simulink model "coif1_7_Level"  (R2021a)
settings: Solver=VariableStepAuto  StartTime=0.0  StopTime=8  RelTol=1e-3
undefined symbols (not defined in the file): lambda2
libraries: dspsigops x15, dspquant2 x1
(part 2 of 4)

== system coif1_7_Level/1st_Level_Decomp/HiD_Even ==
  In_HiD_e : Inport  OutDataTypeStr=double  SampleTime=1/44100
  Add : Sum  AccumDataTypeStr=double  OutDataTypeStr=double  LockScale=on
  Add1 : Sum  AccumDataTypeStr=double  OutDataTypeStr=double  LockScale=on
  Delay{,1..3} (4 alike) : Delay  DelayLength=1  SampleTime=1/44100
  HiD_0 : Constant  Value=0.07273262  OutDataTypeStr=double  SampleTime=1/44100
  HiD_2 : Constant  Value=-0.85257202  OutDataTypeStr=double  SampleTime=1/44100
  HiD_4 : Constant  Value=0.07273262  OutDataTypeStr=double  SampleTime=1/44100
  Multiply : Product  OutDataTypeStr=double  LockScale=on
  Multiply1 : Product  OutDataTypeStr=double  LockScale=on
  Multiply2 : Product  OutDataTypeStr=double  LockScale=on
  Rate Transition : RateTransition  OutPortSampleTime=1/44100
  Rate Transition1 : RateTransition  OutPortSampleTime=1/44100
  Out_HiD_e : Outport  OutDataTypeStr=double  SampleTime=1/44100  VectorParamsAs1DForOutWhenUnconnected=off
  wires:
  In_HiD_e/1 -> Delay/1, Multiply/2
  Delay3/1 -> Add/2
  HiD_2/1 -> Multiply1/1
  Delay/1 -> Rate Transition/1
  Multiply/1 -> Add/1
  Rate Transition/1 -> Delay1/1, Multiply1/2
  HiD_4/1 -> Multiply2/1
  Delay2/1 -> Add1/2
  Multiply1/1 -> Add1/1
  Multiply2/1 -> Delay2/1
  Add1/1 -> Delay3/1
  Rate Transition1/1 -> Multiply2/2
  Add/1 -> Out_HiD_e/1
  Delay1/1 -> Rate Transition1/1
  HiD_0/1 -> Multiply/1

== system coif1_7_Level/1st_Level_Decomp/HiD_Odd ==
  In_HiD_o : Inport  OutDataTypeStr=double  SampleTime=1/44100
  Add : Sum  AccumDataTypeStr=double  OutDataTypeStr=double
  Add1 : Sum  AccumDataTypeStr=double  OutDataTypeStr=double  LockScale=on
  Delay{,1..3} (4 alike) : Delay  DelayLength=1  SampleTime=1/44100
  HiD_1 : Constant  Value=0.337897662  OutDataTypeStr=double  SampleTime=1/44100
  HiD_3 : Constant  Value=0.384864847  OutDataTypeStr=fixdt(1,16,12)  SampleTime=1/44100
  HiD_5 : Constant  Value=-0.015655728  OutDataTypeStr=fixdt(1,16,12)  SampleTime=1/44100
  Multiply : Product  OutDataTypeStr=double  LockScale=on
  Multiply1 : Product  OutDataTypeStr=double  LockScale=on
  Multiply2 : Product  OutDataTypeStr=double  LockScale=on
  Rate Transition : RateTransition  OutPortSampleTime=1/44100
  Rate Transition1 : RateTransition  OutPortSampleTime=1/44100
  Out_HiD_o : Outport  OutDataTypeStr=double  SampleTime=1/44100  VectorParamsAs1DForOutWhenUnconnected=off
  wires:
  In_HiD_o/1 -> Delay/1, Multiply/2
  Delay3/1 -> Add/2
  HiD_3/1 -> Multiply1/1
  Multiply/1 -> Add/1
  Rate Transition/1 -> Delay1/1, Multiply1/2
  Delay2/1 -> Add1/2
  Multiply1/1 -> Add1/1
  Multiply2/1 -> Delay2/1
  Add1/1 -> Delay3/1
  Rate Transition1/1 -> Multiply2/2
  Add/1 -> Out_HiD_o/1
  Delay1/1 -> Rate Transition1/1
  HiD_1/1 -> Multiply/1
  Delay/1 -> Rate Transition/1
  HiD_5/1 -> Multiply2/1

== system coif1_7_Level/1st_Level_Decomp/LoD_Even ==
  In_LoD_e : Inport  OutDataTypeStr=double  SampleTime=1/44100
  Add : Sum  AccumDataTypeStr=double  OutDataTypeStr=double  LockScale=on
  Add1 : Sum  AccumDataTypeStr=double  OutDataTypeStr=double  LockScale=on
  Delay{,1..3} (4 alike) : Delay  DelayLength=1  SampleTime=1/44100
  LoD_0 : Constant  Value=-0.015655728  OutDataTypeStr=double  SampleTime=1/44100
  LoD_2 : Constant  Value=0.384864847  OutDataTypeStr=double  SampleTime=1/44100
  LoD_4 : Constant  Value=0.337897662  OutDataTypeStr=double  SampleTime=1/44100
  Multiply : Product  OutDataTypeStr=double  LockScale=on
  Multiply1 : Product  OutDataTypeStr=double  LockScale=on
  Multiply2 : Product  OutDataTypeStr=double  LockScale=on
  Rate Transition : RateTransition  OutPortSampleTime=1/44100
  Rate Transition1 : RateTransition  OutPortSampleTime=1/44100
  Out_LoD_e : Outport  OutDataTypeStr=double  SampleTime=1/44100  VectorParamsAs1DForOutWhenUnconnected=off
  wires:
  In_LoD_e/1 -> Delay/1, Multiply/2
  Delay3/1 -> Add/2
  LoD_2/1 -> Multiply1/1
  Multiply/1 -> Add/1
  Rate Transition/1 -> Delay1/1, Multiply1/2
  LoD_4/1 -> Multiply2/1
  Delay2/1 -> Add1/2
  Multiply1/1 -> Add1/1
  Multiply2/1 -> Delay2/1
  Add1/1 -> Delay3/1
  Rate Transition1/1 -> Multiply2/2
  Add/1 -> Out_LoD_e/1
  Delay1/1 -> Rate Transition1/1
  LoD_0/1 -> Multiply/1
  Delay/1 -> Rate Transition/1

== system coif1_7_Level/1st_Level_Decomp/LoD_Odd ==
  In_LoD_o : Inport  OutDataTypeStr=double  SampleTime=1/44100
  Add : Sum  AccumDataTypeStr=double  OutDataTypeStr=double  LockScale=on
  Add1 : Sum  AccumDataTypeStr=double  OutDataTypeStr=double  LockScale=on
  Delay{,1..3} (4 alike) : Delay  DelayLength=1  SampleTime=1/44100
  LoD_1 : Constant  Value=-0.07273262  OutDataTypeStr=double  SampleTime=1/44100
  LoD_3 : Constant  Value=0.85257202  OutDataTypeStr=double  SampleTime=1/44100
  LoD_5 : Constant  Value=-0.07273262  OutDataTypeStr=double  SampleTime=1/44100
  Multiply : Product  OutDataTypeStr=double  LockScale=on
  Multiply1 : Product  OutDataTypeStr=double  LockScale=on
  Multiply2 : Product  OutDataTypeStr=double  LockScale=on
  Rate Transition : RateTransition  OutPortSampleTime=1/44100
  Rate Transition1 : RateTransition  OutPortSampleTime=1/44100
  Out_LoD_o : Outport  OutDataTypeStr=double  SampleTime=1/44100  VectorParamsAs1DForOutWhenUnconnected=off
  wires:
  In_LoD_o/1 -> Delay/1, Multiply/2
  Delay3/1 -> Add/2
  LoD_3/1 -> Multiply1/1
  Delay/1 -> Rate Transition/1
  Multiply/1 -> Add/1
  Rate Transition/1 -> Delay1/1, Multiply1/2
  LoD_5/1 -> Multiply2/1
  Delay2/1 -> Add1/2
  Multiply1/1 -> Add1/1
  Multiply2/1 -> Delay2/1
  Add1/1 -> Delay3/1
  Rate Transition1/1 -> Multiply2/2
  Add/1 -> Out_LoD_o/1
  Delay1/1 -> Rate Transition1/1
  LoD_1/1 -> Multiply/1

== system coif1_7_Level/1st_Level_Recon/HiR_Even1 ==
  In_HiR_e : Inport  OutDataTypeStr=double  SampleTime=1/44100
  Add : Sum  AccumDataTypeStr=double  OutDataTypeStr=double  LockScale=on
  Add1 : Sum  AccumDataTypeStr=double  OutDataTypeStr=double  LockScale=on
  Delay{,1..3} (4 alike) : Delay  DelayLength=1  SampleTime=1/44100
  HiR_0 : Constant  Value=-0.015655728  OutDataTypeStr=double  SampleTime=1/44100
  HiR_2 : Constant  Value=0.384864847  OutDataTypeStr=double  SampleTime=1/44100
  HiR_4 : Constant  Value=0.337897662  OutDataTypeStr=double  SampleTime=1/44100
  Multiply : Product  OutDataTypeStr=double  LockScale=on
  Multiply1 : Product  OutDataTypeStr=double  LockScale=on
  Multiply2 : Product  OutDataTypeStr=double  LockScale=on
  Rate Transition : RateTransition  OutPortSampleTime=1/44100
  Rate Transition1 : RateTransition  OutPortSampleTime=1/44100
  Out_HiR_e : Outport  OutDataTypeStr=double  SampleTime=1/44100  VectorParamsAs1DForOutWhenUnconnected=off
  wires:
  In_HiR_e/1 -> Multiply/2, Delay/1
  Delay/1 -> Rate Transition/1
  Delay3/1 -> Add/2
  Multiply/1 -> Add/1
  HiR_0/1 -> Multiply/1
  HiR_2/1 -> Multiply1/1
  Rate Transition/1 -> Delay1/1, Multiply1/2
  Add/1 -> Out_HiR_e/1
  Delay1/1 -> Rate Transition1/1
  Rate Transition1/1 -> Multiply2/2
  Multiply2/1 -> Delay2/1
  Delay2/1 -> Add1/2
  Multiply1/1 -> Add1/1
  Add1/1 -> Delay3/1
  HiR_4/1 -> Multiply2/1

== system coif1_7_Level/1st_Level_Recon/HiR_Odd1 ==
  In_HiR_o : Inport  OutDataTypeStr=double  SampleTime=1/44100
  Add1 : Sum  AccumDataTypeStr=double  OutDataTypeStr=double  LockScale=on
  Add2 : Sum  AccumDataTypeStr=double  OutDataTypeStr=double  LockScale=on
  Delay{1..2,4..5} (4 alike) : Delay  DelayLength=1  SampleTime=1/44100
  HiR_1 : Constant  Value=0.07273262  OutDataTypeStr=double  SampleTime=1/44100
  HiR_3 : Constant  Value=-0.85257202  OutDataTypeStr=double  SampleTime=1/44100
  HiR_5 : Constant  Value=0.07273262  OutDataTypeStr=double  SampleTime=1/44100
  Multiply2 : Product  OutDataTypeStr=double  LockScale=on
  Multiply3 : Product  OutDataTypeStr=double  LockScale=on
  Multiply4 : Product  OutDataTypeStr=double  LockScale=on
  Rate Transition1 : RateTransition  OutPortSampleTime=1/44100
  Rate Transition2 : RateTransition  OutPortSampleTime=1/44100
  Out_HiR_o : Outport  OutDataTypeStr=double  SampleTime=1/44100  VectorParamsAs1DForOutWhenUnconnected=off
  wires:
  HiR_5/1 -> Multiply4/1
  Add1/1 -> Out_HiR_o/1
  Rate Transition2/1 -> Multiply4/2
  Rate Transition1/1 -> Delay2/1, Multiply3/2
  Multiply4/1 -> Delay4/1
  Add2/1 -> Delay5/1
  Multiply3/1 -> Add2/1
  Delay4/1 -> Add2/2
  Multiply2/1 -> Add1/1
  Delay2/1 -> Rate Transition2/1
  In_HiR_o/1 -> Multiply2/2, Delay1/1
  Delay1/1 -> Rate Transition1/1
  Delay5/1 -> Add1/2
  HiR_1/1 -> Multiply2/1
  HiR_3/1 -> Multiply3/1

== system coif1_7_Level/1st_Level_Recon/LoR_Even1 ==
  In_LoR_e : Inport  OutDataTypeStr=double  SampleTime=1/44100
  Add1 : Sum  AccumDataTypeStr=double  OutDataTypeStr=double  LockScale=on
  Add2 : Sum  AccumDataTypeStr=double  OutDataTypeStr=double  LockScale=on
  Delay{1..2,4..5} (4 alike) : Delay  DelayLength=1  SampleTime=1/44100
  LoR_0 : Constant  Value=-0.07273262  OutDataTypeStr=double  SampleTime=1/44100
  LoR_2 : Constant  Value=0.85257202  OutDataTypeStr=double  SampleTime=1/44100
  LoR_4 : Constant  Value=-0.07273262  OutDataTypeStr=double  SampleTime=1/44100
  Multiply2 : Product  OutDataTypeStr=double  LockScale=on
  Multiply3 : Product  OutDataTypeStr=double  LockScale=on
  Multiply4 : Product  OutDataTypeStr=double  LockScale=on
  Rate Transition1 : RateTransition  OutPortSampleTime=1/44100
  Rate Transition2 : RateTransition  OutPortSampleTime=1/44100
  Out_LoR_e : Outport  OutDataTypeStr=double  SampleTime=1/44100  VectorParamsAs1DForOutWhenUnconnected=off
  wires:
  Add2/1 -> Delay5/1
  Delay2/1 -> Rate Transition2/1
  Add1/1 -> Out_LoR_e/1
  Multiply3/1 -> Add2/1
  Delay5/1 -> Add1/2
  Delay1/1 -> Rate Transition1/1
  Multiply2/1 -> Add1/1
  Delay4/1 -> Add2/2
  Multiply4/1 -> Delay4/1
  Rate Transition2/1 -> Multiply4/2
  In_LoR_e/1 -> Multiply2/2, Delay1/1
  Rate Transition1/1 -> Delay2/1, Multiply3/2
  LoR_4/1 -> Multiply4/1
  LoR_2/1 -> Multiply3/1
  LoR_0/1 -> Multiply2/1

== system coif1_7_Level/1st_Level_Recon/LoR_Odd1 ==
  In_LoR_o : Inport  OutDataTypeStr=double  SampleTime=1/44100
  Add1 : Sum  AccumDataTypeStr=double  OutDataTypeStr=double  LockScale=on
  Add2 : Sum  AccumDataTypeStr=double  OutDataTypeStr=double  LockScale=on
  Delay{1..2,4..5} (4 alike) : Delay  DelayLength=1  SampleTime=1/44100
  LoR_1 : Constant  Value=0.337897662  OutDataTypeStr=double  SampleTime=1/44100
  LoR_3 : Constant  Value=0.384864847  OutDataTypeStr=double  SampleTime=1/44100
  LoR_5 : Constant  Value=-0.015655728  OutDataTypeStr=double  SampleTime=1/44100
  Multiply2 : Product  OutDataTypeStr=double  LockScale=on
  Multiply3 : Product  OutDataTypeStr=double  LockScale=on
  Multiply4 : Product  OutDataTypeStr=double  LockScale=on
  Rate Transition1 : RateTransition  OutPortSampleTime=1/44100
  Rate Transition2 : RateTransition  OutPortSampleTime=1/44100
  Out_HiR_o : Outport  OutDataTypeStr=double  SampleTime=1/44100  VectorParamsAs1DForOutWhenUnconnected=off
  wires:
  LoR_5/1 -> Multiply4/1
  In_LoR_o/1 -> Multiply2/2, Delay1/1
  LoR_3/1 -> Multiply3/1
  Delay2/1 -> Rate Transition2/1
  Add2/1 -> Delay5/1
  Multiply3/1 -> Add2/1
  Multiply2/1 -> Add1/1
  Delay4/1 -> Add2/2
  Rate Transition1/1 -> Delay2/1, Multiply3/2
  LoR_1/1 -> Multiply2/1
  Delay5/1 -> Add1/2
  Rate Transition2/1 -> Multiply4/2
  Delay1/1 -> Rate Transition1/1
  Multiply4/1 -> Delay4/1
  Add1/1 -> Out_HiR_o/1

== system coif1_7_Level/2nd_Level_Decomp/HiD_Even ==
  In_HiD_e : Inport  OutDataTypeStr=double  SampleTime=1/44100
  Add : Sum  AccumDataTypeStr=double  OutDataTypeStr=double  LockScale=on
  Add1 : Sum  AccumDataTypeStr=double  OutDataTypeStr=double  LockScale=on
  Delay{,1..3} (4 alike) : Delay  DelayLength=1  SampleTime=1/44100
  HiD_0 : Constant  Value=0.07273262  OutDataTypeStr=double  SampleTime=1/44100
  HiD_2 : Constant  Value=-0.85257202  OutDataTypeStr=double  SampleTime=1/44100
  HiD_4 : Constant  Value=0.07273262  OutDataTypeStr=double  SampleTime=1/44100
  Multiply : Product  OutDataTypeStr=double  LockScale=on
  Multiply1 : Product  OutDataTypeStr=double  LockScale=on
  Multiply2 : Product  OutDataTypeStr=double  LockScale=on
  Rate Transition : RateTransition  OutPortSampleTime=1/44100
  Rate Transition1 : RateTransition  OutPortSampleTime=1/44100
  Out_HiD_e : Outport  OutDataTypeStr=double  SampleTime=1/44100  VectorParamsAs1DForOutWhenUnconnected=off
  wires:
  In_HiD_e/1 -> Delay/1, Multiply/2
  Delay3/1 -> Add/2
  HiD_2/1 -> Multiply1/1
  Delay/1 -> Rate Transition/1
  Multiply/1 -> Add/1
  Rate Transition/1 -> Delay1/1, Multiply1/2
  HiD_4/1 -> Multiply2/1
  Delay2/1 -> Add1/2
  Multiply1/1 -> Add1/1
  Multiply2/1 -> Delay2/1
  Add1/1 -> Delay3/1
  Rate Transition1/1 -> Multiply2/2
  Add/1 -> Out_HiD_e/1
  Delay1/1 -> Rate Transition1/1
  HiD_0/1 -> Multiply/1

== system coif1_7_Level/2nd_Level_Decomp/HiD_Odd ==
  In_HiD_o : Inport  OutDataTypeStr=double  SampleTime=1/44100
  Add : Sum  AccumDataTypeStr=double  OutDataTypeStr=double
  Add1 : Sum  AccumDataTypeStr=double  OutDataTypeStr=double  LockScale=on
  Delay{,1..3} (4 alike) : Delay  DelayLength=1  SampleTime=1/44100
  HiD_1 : Constant  Value=0.337897662  OutDataTypeStr=double  SampleTime=1/44100
  HiD_3 : Constant  Value=0.384864847  OutDataTypeStr=fixdt(1,16,12)  SampleTime=1/44100
  HiD_5 : Constant  Value=-0.015655728  OutDataTypeStr=fixdt(1,16,12)  SampleTime=1/44100
  Multiply : Product  OutDataTypeStr=double  LockScale=on
  Multiply1 : Product  OutDataTypeStr=double  LockScale=on
  Multiply2 : Product  OutDataTypeStr=double  LockScale=on
  Rate Transition : RateTransition  OutPortSampleTime=1/44100
  Rate Transition1 : RateTransition  OutPortSampleTime=1/44100
  Out_HiD_o : Outport  OutDataTypeStr=double  SampleTime=1/44100  VectorParamsAs1DForOutWhenUnconnected=off
  wires:
  In_HiD_o/1 -> Delay/1, Multiply/2
  Delay3/1 -> Add/2
  HiD_3/1 -> Multiply1/1
  Multiply/1 -> Add/1
  Rate Transition/1 -> Delay1/1, Multiply1/2
  Delay2/1 -> Add1/2
  Multiply1/1 -> Add1/1
  Multiply2/1 -> Delay2/1
  Add1/1 -> Delay3/1
  Rate Transition1/1 -> Multiply2/2
  Add/1 -> Out_HiD_o/1
  Delay1/1 -> Rate Transition1/1
  HiD_1/1 -> Multiply/1
  Delay/1 -> Rate Transition/1
  HiD_5/1 -> Multiply2/1

== system coif1_7_Level/2nd_Level_Decomp/LoD_Even ==
  In_LoD_e : Inport  OutDataTypeStr=double  SampleTime=1/44100
  Add : Sum  AccumDataTypeStr=double  OutDataTypeStr=double  LockScale=on
  Add1 : Sum  AccumDataTypeStr=double  OutDataTypeStr=double  LockScale=on
  Delay{,1..3} (4 alike) : Delay  DelayLength=1  SampleTime=1/44100
  LoD_0 : Constant  Value=-0.015655728  OutDataTypeStr=double  SampleTime=1/44100
  LoD_2 : Constant  Value=0.384864847  OutDataTypeStr=double  SampleTime=1/44100
  LoD_4 : Constant  Value=0.337897662  OutDataTypeStr=double  SampleTime=1/44100
  Multiply : Product  OutDataTypeStr=double  LockScale=on
  Multiply1 : Product  OutDataTypeStr=double  LockScale=on
  Multiply2 : Product  OutDataTypeStr=double  LockScale=on
  Rate Transition : RateTransition  OutPortSampleTime=1/44100
  Rate Transition1 : RateTransition  OutPortSampleTime=1/44100
  Out_LoD_e : Outport  OutDataTypeStr=double  SampleTime=1/44100  VectorParamsAs1DForOutWhenUnconnected=off
  wires:
  In_LoD_e/1 -> Delay/1, Multiply/2
  Delay3/1 -> Add/2
  LoD_2/1 -> Multiply1/1
  Multiply/1 -> Add/1
  Rate Transition/1 -> Delay1/1, Multiply1/2
  LoD_4/1 -> Multiply2/1
  Delay2/1 -> Add1/2
  Multiply1/1 -> Add1/1
  Multiply2/1 -> Delay2/1
  Add1/1 -> Delay3/1
  Rate Transition1/1 -> Multiply2/2
  Add/1 -> Out_LoD_e/1
  Delay1/1 -> Rate Transition1/1
  LoD_0/1 -> Multiply/1
  Delay/1 -> Rate Transition/1

== system coif1_7_Level/2nd_Level_Decomp/LoD_Odd ==
  In_LoD_o : Inport  OutDataTypeStr=double  SampleTime=1/44100
  Add : Sum  AccumDataTypeStr=double  OutDataTypeStr=double  LockScale=on
  Add1 : Sum  AccumDataTypeStr=double  OutDataTypeStr=double  LockScale=on
  Delay{,1..3} (4 alike) : Delay  DelayLength=1  SampleTime=1/44100
  LoD_1 : Constant  Value=-0.07273262  OutDataTypeStr=double  SampleTime=1/44100
  LoD_3 : Constant  Value=0.85257202  OutDataTypeStr=double  SampleTime=1/44100
  LoD_5 : Constant  Value=-0.07273262  OutDataTypeStr=double  SampleTime=1/44100
  Multiply : Product  OutDataTypeStr=double  LockScale=on
  Multiply1 : Product  OutDataTypeStr=double  LockScale=on
  Multiply2 : Product  OutDataTypeStr=double  LockScale=on
  Rate Transition : RateTransition  OutPortSampleTime=1/44100
  Rate Transition1 : RateTransition  OutPortSampleTime=1/44100
  Out_LoD_o : Outport  OutDataTypeStr=double  SampleTime=1/44100  VectorParamsAs1DForOutWhenUnconnected=off
  wires:
  In_LoD_o/1 -> Delay/1, Multiply/2
  Delay3/1 -> Add/2
  LoD_3/1 -> Multiply1/1
  Delay/1 -> Rate Transition/1
  Multiply/1 -> Add/1
  Rate Transition/1 -> Delay1/1, Multiply1/2
  LoD_5/1 -> Multiply2/1
  Delay2/1 -> Add1/2
  Multiply1/1 -> Add1/1
  Multiply2/1 -> Delay2/1
  Add1/1 -> Delay3/1
  Rate Transition1/1 -> Multiply2/2
  Add/1 -> Out_LoD_o/1
  Delay1/1 -> Rate Transition1/1
  LoD_1/1 -> Multiply/1

== system coif1_7_Level/2nd_Level_Recon/HiR_Even1 ==
  In_HiR_e : Inport  OutDataTypeStr=double  SampleTime=1/44100
  Add : Sum  AccumDataTypeStr=double  OutDataTypeStr=double  LockScale=on
  Add1 : Sum  AccumDataTypeStr=double  OutDataTypeStr=double  LockScale=on
  Delay{,1..3} (4 alike) : Delay  DelayLength=1  SampleTime=1/44100
  HiR_0 : Constant  Value=-0.015655728  OutDataTypeStr=double  SampleTime=1/44100
  HiR_2 : Constant  Value=0.384864847  OutDataTypeStr=double  SampleTime=1/44100
  HiR_4 : Constant  Value=0.337897662  OutDataTypeStr=double  SampleTime=1/44100
  Multiply : Product  OutDataTypeStr=double  LockScale=on
  Multiply1 : Product  OutDataTypeStr=double  LockScale=on
  Multiply2 : Product  OutDataTypeStr=double  LockScale=on
  Rate Transition : RateTransition  OutPortSampleTime=1/44100
  Rate Transition1 : RateTransition  OutPortSampleTime=1/44100
  Out_HiR_e : Outport  OutDataTypeStr=double  SampleTime=1/44100  VectorParamsAs1DForOutWhenUnconnected=off
  wires:
  In_HiR_e/1 -> Multiply/2, Delay/1
  Delay/1 -> Rate Transition/1
  Delay3/1 -> Add/2
  Multiply/1 -> Add/1
  HiR_0/1 -> Multiply/1
  HiR_2/1 -> Multiply1/1
  Rate Transition/1 -> Delay1/1, Multiply1/2
  Add/1 -> Out_HiR_e/1
  Delay1/1 -> Rate Transition1/1
  Rate Transition1/1 -> Multiply2/2
  Multiply2/1 -> Delay2/1
  Delay2/1 -> Add1/2
  Multiply1/1 -> Add1/1
  Add1/1 -> Delay3/1
  HiR_4/1 -> Multiply2/1

== system coif1_7_Level/2nd_Level_Recon/HiR_Odd1 ==
  In_HiR_o : Inport  OutDataTypeStr=double  SampleTime=1/44100
  Add1 : Sum  AccumDataTypeStr=double  OutDataTypeStr=double  LockScale=on
  Add2 : Sum  AccumDataTypeStr=double  OutDataTypeStr=double  LockScale=on
  Delay{1..2,4..5} (4 alike) : Delay  DelayLength=1  SampleTime=1/44100
  HiR_1 : Constant  Value=0.07273262  OutDataTypeStr=double  SampleTime=1/44100
  HiR_3 : Constant  Value=-0.85257202  OutDataTypeStr=double  SampleTime=1/44100
  HiR_5 : Constant  Value=0.07273262  OutDataTypeStr=double  SampleTime=1/44100
  Multiply2 : Product  OutDataTypeStr=double  LockScale=on
  Multiply3 : Product  OutDataTypeStr=double  LockScale=on
  Multiply4 : Product  OutDataTypeStr=double  LockScale=on
  Rate Transition1 : RateTransition  OutPortSampleTime=1/44100
  Rate Transition2 : RateTransition  OutPortSampleTime=1/44100
  Out_HiR_o : Outport  OutDataTypeStr=double  SampleTime=1/44100  VectorParamsAs1DForOutWhenUnconnected=off
  wires:
  HiR_5/1 -> Multiply4/1
  Add1/1 -> Out_HiR_o/1
  Rate Transition2/1 -> Multiply4/2
  Rate Transition1/1 -> Delay2/1, Multiply3/2
  Multiply4/1 -> Delay4/1
  Add2/1 -> Delay5/1
  Multiply3/1 -> Add2/1
  Delay4/1 -> Add2/2
  Multiply2/1 -> Add1/1
  Delay2/1 -> Rate Transition2/1
  In_HiR_o/1 -> Multiply2/2, Delay1/1
  Delay1/1 -> Rate Transition1/1
  Delay5/1 -> Add1/2
  HiR_1/1 -> Multiply2/1
  HiR_3/1 -> Multiply3/1

== system coif1_7_Level/2nd_Level_Recon/LoR_Even1 ==
  In_LoR_e : Inport  OutDataTypeStr=double  SampleTime=1/44100
  Add1 : Sum  AccumDataTypeStr=double  OutDataTypeStr=double  LockScale=on
  Add2 : Sum  AccumDataTypeStr=double  OutDataTypeStr=double  LockScale=on
  Delay{1..2,4..5} (4 alike) : Delay  DelayLength=1  SampleTime=1/44100
  LoR_0 : Constant  Value=-0.07273262  OutDataTypeStr=double  SampleTime=1/44100
  LoR_2 : Constant  Value=0.85257202  OutDataTypeStr=double  SampleTime=1/44100
  LoR_4 : Constant  Value=-0.07273262  OutDataTypeStr=double  SampleTime=1/44100
  Multiply2 : Product  OutDataTypeStr=double  LockScale=on
  Multiply3 : Product  OutDataTypeStr=double  LockScale=on
  Multiply4 : Product  OutDataTypeStr=double  LockScale=on
  Rate Transition1 : RateTransition  OutPortSampleTime=1/44100
  Rate Transition2 : RateTransition  OutPortSampleTime=1/44100
  Out_LoR_e : Outport  OutDataTypeStr=double  SampleTime=1/44100  VectorParamsAs1DForOutWhenUnconnected=off
  wires:
  Add2/1 -> Delay5/1
  Delay2/1 -> Rate Transition2/1
  Add1/1 -> Out_LoR_e/1
  Multiply3/1 -> Add2/1
  Delay5/1 -> Add1/2
  Delay1/1 -> Rate Transition1/1
  Multiply2/1 -> Add1/1
  Delay4/1 -> Add2/2
  Multiply4/1 -> Delay4/1
  Rate Transition2/1 -> Multiply4/2
  In_LoR_e/1 -> Multiply2/2, Delay1/1
  Rate Transition1/1 -> Delay2/1, Multiply3/2
  LoR_4/1 -> Multiply4/1
  LoR_2/1 -> Multiply3/1
  LoR_0/1 -> Multiply2/1

== system coif1_7_Level/2nd_Level_Recon/LoR_Odd1 ==
  In_LoR_o : Inport  OutDataTypeStr=double  SampleTime=1/44100
  Add1 : Sum  AccumDataTypeStr=double  OutDataTypeStr=double  LockScale=on
  Add2 : Sum  AccumDataTypeStr=double  OutDataTypeStr=double  LockScale=on
  Delay{1..2,4..5} (4 alike) : Delay  DelayLength=1  SampleTime=1/44100
  LoR_1 : Constant  Value=0.337897662  OutDataTypeStr=double  SampleTime=1/44100
  LoR_3 : Constant  Value=0.384864847  OutDataTypeStr=double  SampleTime=1/44100
  LoR_5 : Constant  Value=-0.015655728  OutDataTypeStr=double  SampleTime=1/44100
  Multiply2 : Product  OutDataTypeStr=double  LockScale=on
  Multiply3 : Product  OutDataTypeStr=double  LockScale=on
  Multiply4 : Product  OutDataTypeStr=double  LockScale=on
  Rate Transition1 : RateTransition  OutPortSampleTime=1/44100
  Rate Transition2 : RateTransition  OutPortSampleTime=1/44100
  Out_HiR_o : Outport  OutDataTypeStr=double  SampleTime=1/44100  VectorParamsAs1DForOutWhenUnconnected=off
  wires:
  LoR_5/1 -> Multiply4/1
  In_LoR_o/1 -> Multiply2/2, Delay1/1
  LoR_3/1 -> Multiply3/1
  Delay2/1 -> Rate Transition2/1
  Add2/1 -> Delay5/1
  Multiply3/1 -> Add2/1
  Multiply2/1 -> Add1/1
  Delay4/1 -> Add2/2
  Rate Transition1/1 -> Delay2/1, Multiply3/2
  LoR_1/1 -> Multiply2/1
  Delay5/1 -> Add1/2
  Rate Transition2/1 -> Multiply4/2
  Delay1/1 -> Rate Transition1/1
  Multiply4/1 -> Delay4/1
  Add1/1 -> Out_HiR_o/1

== system coif1_7_Level/3rd_Level_Decomp/HiD_Even ==
  In_HiD_e : Inport  OutDataTypeStr=double  SampleTime=1/44100
  Add : Sum  AccumDataTypeStr=double  OutDataTypeStr=double  LockScale=on
  Add1 : Sum  AccumDataTypeStr=double  OutDataTypeStr=double  LockScale=on
  Delay{,1..3} (4 alike) : Delay  DelayLength=1  SampleTime=1/44100
  HiD_0 : Constant  Value=0.07273262  OutDataTypeStr=double  SampleTime=1/44100
  HiD_2 : Constant  Value=-0.85257202  OutDataTypeStr=double  SampleTime=1/44100
  HiD_4 : Constant  Value=0.07273262  OutDataTypeStr=double  SampleTime=1/44100
  Multiply : Product  OutDataTypeStr=double  LockScale=on
  Multiply1 : Product  OutDataTypeStr=double  LockScale=on
  Multiply2 : Product  OutDataTypeStr=double  LockScale=on
  Rate Transition : RateTransition  OutPortSampleTime=1/44100
  Rate Transition1 : RateTransition  OutPortSampleTime=1/44100
  Out_HiD_e : Outport  OutDataTypeStr=double  SampleTime=1/44100  VectorParamsAs1DForOutWhenUnconnected=off
  wires:
  In_HiD_e/1 -> Delay/1, Multiply/2
  Delay3/1 -> Add/2
  HiD_2/1 -> Multiply1/1
  Delay/1 -> Rate Transition/1
  Multiply/1 -> Add/1
  Rate Transition/1 -> Delay1/1, Multiply1/2
  HiD_4/1 -> Multiply2/1
  Delay2/1 -> Add1/2
  Multiply1/1 -> Add1/1
  Multiply2/1 -> Delay2/1
  Add1/1 -> Delay3/1
  Rate Transition1/1 -> Multiply2/2
  Add/1 -> Out_HiD_e/1
  Delay1/1 -> Rate Transition1/1
  HiD_0/1 -> Multiply/1

== system coif1_7_Level/3rd_Level_Decomp/HiD_Odd ==
  In_HiD_o : Inport  OutDataTypeStr=double  SampleTime=1/44100
  Add : Sum  AccumDataTypeStr=double  OutDataTypeStr=double
  Add1 : Sum  AccumDataTypeStr=double  OutDataTypeStr=double  LockScale=on
  Delay{,1..3} (4 alike) : Delay  DelayLength=1  SampleTime=1/44100
  HiD_1 : Constant  Value=0.337897662  OutDataTypeStr=double  SampleTime=1/44100
  HiD_3 : Constant  Value=0.384864847  OutDataTypeStr=fixdt(1,16,12)  SampleTime=1/44100
  HiD_5 : Constant  Value=-0.015655728  OutDataTypeStr=fixdt(1,16,12)  SampleTime=1/44100
  Multiply : Product  OutDataTypeStr=double  LockScale=on
  Multiply1 : Product  OutDataTypeStr=double  LockScale=on
  Multiply2 : Product  OutDataTypeStr=double  LockScale=on
  Rate Transition : RateTransition  OutPortSampleTime=1/44100
  Rate Transition1 : RateTransition  OutPortSampleTime=1/44100
  Out_HiD_o : Outport  OutDataTypeStr=double  SampleTime=1/44100  VectorParamsAs1DForOutWhenUnconnected=off
  wires:
  In_HiD_o/1 -> Delay/1, Multiply/2
  Delay3/1 -> Add/2
  HiD_3/1 -> Multiply1/1
  Multiply/1 -> Add/1
  Rate Transition/1 -> Delay1/1, Multiply1/2
  Delay2/1 -> Add1/2
  Multiply1/1 -> Add1/1
  Multiply2/1 -> Delay2/1
  Add1/1 -> Delay3/1
  Rate Transition1/1 -> Multiply2/2
  Add/1 -> Out_HiD_o/1
  Delay1/1 -> Rate Transition1/1
  HiD_1/1 -> Multiply/1
  Delay/1 -> Rate Transition/1
  HiD_5/1 -> Multiply2/1

== system coif1_7_Level/3rd_Level_Decomp/LoD_Even ==
  In_LoD_e : Inport  OutDataTypeStr=double  SampleTime=1/44100
  Add : Sum  AccumDataTypeStr=double  OutDataTypeStr=double  LockScale=on
  Add1 : Sum  AccumDataTypeStr=double  OutDataTypeStr=double  LockScale=on
  Delay{,1..3} (4 alike) : Delay  DelayLength=1  SampleTime=1/44100
  LoD_0 : Constant  Value=-0.015655728  OutDataTypeStr=double  SampleTime=1/44100
  LoD_2 : Constant  Value=0.384864847  OutDataTypeStr=double  SampleTime=1/44100
  LoD_4 : Constant  Value=0.337897662  OutDataTypeStr=double  SampleTime=1/44100
  Multiply : Product  OutDataTypeStr=double  LockScale=on
  Multiply1 : Product  OutDataTypeStr=double  LockScale=on
  Multiply2 : Product  OutDataTypeStr=double  LockScale=on
  Rate Transition : RateTransition  OutPortSampleTime=1/44100
  Rate Transition1 : RateTransition  OutPortSampleTime=1/44100
  Out_LoD_e : Outport  OutDataTypeStr=double  SampleTime=1/44100  VectorParamsAs1DForOutWhenUnconnected=off
  wires:
  In_LoD_e/1 -> Delay/1, Multiply/2
  Delay3/1 -> Add/2
  LoD_2/1 -> Multiply1/1
  Multiply/1 -> Add/1
  Rate Transition/1 -> Delay1/1, Multiply1/2
  LoD_4/1 -> Multiply2/1
  Delay2/1 -> Add1/2
  Multiply1/1 -> Add1/1
  Multiply2/1 -> Delay2/1
  Add1/1 -> Delay3/1
  Rate Transition1/1 -> Multiply2/2
  Add/1 -> Out_LoD_e/1
  Delay1/1 -> Rate Transition1/1
  LoD_0/1 -> Multiply/1
  Delay/1 -> Rate Transition/1

== system coif1_7_Level/3rd_Level_Decomp/LoD_Odd ==
  In_LoD_o : Inport  OutDataTypeStr=double  SampleTime=1/44100
  Add : Sum  AccumDataTypeStr=double  OutDataTypeStr=double  LockScale=on
  Add1 : Sum  AccumDataTypeStr=double  OutDataTypeStr=double  LockScale=on
  Delay{,1..3} (4 alike) : Delay  DelayLength=1  SampleTime=1/44100
  LoD_1 : Constant  Value=-0.07273262  OutDataTypeStr=double  SampleTime=1/44100
  LoD_3 : Constant  Value=0.85257202  OutDataTypeStr=double  SampleTime=1/44100
  LoD_5 : Constant  Value=-0.07273262  OutDataTypeStr=double  SampleTime=1/44100
  Multiply : Product  OutDataTypeStr=double  LockScale=on
  Multiply1 : Product  OutDataTypeStr=double  LockScale=on
  Multiply2 : Product  OutDataTypeStr=double  LockScale=on
  Rate Transition : RateTransition  OutPortSampleTime=1/44100
  Rate Transition1 : RateTransition  OutPortSampleTime=1/44100
  Out_LoD_o : Outport  OutDataTypeStr=double  SampleTime=1/44100  VectorParamsAs1DForOutWhenUnconnected=off
  wires:
  In_LoD_o/1 -> Delay/1, Multiply/2
  Delay3/1 -> Add/2
  LoD_3/1 -> Multiply1/1
  Delay/1 -> Rate Transition/1
  Multiply/1 -> Add/1
  Rate Transition/1 -> Delay1/1, Multiply1/2
  LoD_5/1 -> Multiply2/1
  Delay2/1 -> Add1/2
  Multiply1/1 -> Add1/1
  Multiply2/1 -> Delay2/1
  Add1/1 -> Delay3/1
  Rate Transition1/1 -> Multiply2/2
  Add/1 -> Out_LoD_o/1
  Delay1/1 -> Rate Transition1/1
  LoD_1/1 -> Multiply/1

== system coif1_7_Level/3rd_Level_Recon/HiR_Even1 ==
  In_HiR_e : Inport  OutDataTypeStr=double  SampleTime=1/44100
  Add : Sum  AccumDataTypeStr=double  OutDataTypeStr=double  LockScale=on
  Add1 : Sum  AccumDataTypeStr=double  OutDataTypeStr=double  LockScale=on
  Delay{,1..3} (4 alike) : Delay  DelayLength=1  SampleTime=1/44100
  HiR_0 : Constant  Value=-0.015655728  OutDataTypeStr=double  SampleTime=1/44100
  HiR_2 : Constant  Value=0.384864847  OutDataTypeStr=double  SampleTime=1/44100
  HiR_4 : Constant  Value=0.337897662  OutDataTypeStr=double  SampleTime=1/44100
  Multiply : Product  OutDataTypeStr=double  LockScale=on
  Multiply1 : Product  OutDataTypeStr=double  LockScale=on
  Multiply2 : Product  OutDataTypeStr=double  LockScale=on
  Rate Transition : RateTransition  OutPortSampleTime=1/44100
  Rate Transition1 : RateTransition  OutPortSampleTime=1/44100
  Out_HiR_e : Outport  OutDataTypeStr=double  SampleTime=1/44100  VectorParamsAs1DForOutWhenUnconnected=off
  wires:
  In_HiR_e/1 -> Multiply/2, Delay/1
  Delay/1 -> Rate Transition/1
  Delay3/1 -> Add/2
  Multiply/1 -> Add/1
  HiR_0/1 -> Multiply/1
  HiR_2/1 -> Multiply1/1
  Rate Transition/1 -> Delay1/1, Multiply1/2
  Add/1 -> Out_HiR_e/1
  Delay1/1 -> Rate Transition1/1
  Rate Transition1/1 -> Multiply2/2
  Multiply2/1 -> Delay2/1
  Delay2/1 -> Add1/2
  Multiply1/1 -> Add1/1
  Add1/1 -> Delay3/1
  HiR_4/1 -> Multiply2/1

== system coif1_7_Level/3rd_Level_Recon/HiR_Odd1 ==
  In_HiR_o : Inport  OutDataTypeStr=double  SampleTime=1/44100
  Add1 : Sum  AccumDataTypeStr=double  OutDataTypeStr=double  LockScale=on
  Add2 : Sum  AccumDataTypeStr=double  OutDataTypeStr=double  LockScale=on
  Delay{1..2,4..5} (4 alike) : Delay  DelayLength=1  SampleTime=1/44100
  HiR_1 : Constant  Value=0.07273262  OutDataTypeStr=double  SampleTime=1/44100
  HiR_3 : Constant  Value=-0.85257202  OutDataTypeStr=double  SampleTime=1/44100
  HiR_5 : Constant  Value=0.07273262  OutDataTypeStr=double  SampleTime=1/44100
  Multiply2 : Product  OutDataTypeStr=double  LockScale=on
  Multiply3 : Product  OutDataTypeStr=double  LockScale=on
  Multiply4 : Product  OutDataTypeStr=double  LockScale=on
  Rate Transition1 : RateTransition  OutPortSampleTime=1/44100
  Rate Transition2 : RateTransition  OutPortSampleTime=1/44100
  Out_HiR_o : Outport  OutDataTypeStr=double  SampleTime=1/44100  VectorParamsAs1DForOutWhenUnconnected=off
  wires:
  HiR_5/1 -> Multiply4/1
  Add1/1 -> Out_HiR_o/1
  Rate Transition2/1 -> Multiply4/2
  Rate Transition1/1 -> Delay2/1, Multiply3/2
  Multiply4/1 -> Delay4/1
  Add2/1 -> Delay5/1
  Multiply3/1 -> Add2/1
  Delay4/1 -> Add2/2
  Multiply2/1 -> Add1/1
  Delay2/1 -> Rate Transition2/1
  In_HiR_o/1 -> Multiply2/2, Delay1/1
  Delay1/1 -> Rate Transition1/1
  Delay5/1 -> Add1/2
  HiR_1/1 -> Multiply2/1
  HiR_3/1 -> Multiply3/1

== system coif1_7_Level/3rd_Level_Recon/LoR_Even1 ==
  In_LoR_e : Inport  OutDataTypeStr=double  SampleTime=1/44100
  Add1 : Sum  AccumDataTypeStr=double  OutDataTypeStr=double  LockScale=on
  Add2 : Sum  AccumDataTypeStr=double  OutDataTypeStr=double  LockScale=on
  Delay{1..2,4..5} (4 alike) : Delay  DelayLength=1  SampleTime=1/44100
  LoR_0 : Constant  Value=-0.07273262  OutDataTypeStr=double  SampleTime=1/44100
  LoR_2 : Constant  Value=0.85257202  OutDataTypeStr=double  SampleTime=1/44100
  LoR_4 : Constant  Value=-0.07273262  OutDataTypeStr=double  SampleTime=1/44100
  Multiply2 : Product  OutDataTypeStr=double  LockScale=on
  Multiply3 : Product  OutDataTypeStr=double  LockScale=on
  Multiply4 : Product  OutDataTypeStr=double  LockScale=on
  Rate Transition1 : RateTransition  OutPortSampleTime=1/44100
  Rate Transition2 : RateTransition  OutPortSampleTime=1/44100
  Out_LoR_e : Outport  OutDataTypeStr=double  SampleTime=1/44100  VectorParamsAs1DForOutWhenUnconnected=off
  wires:
  Add2/1 -> Delay5/1
  Delay2/1 -> Rate Transition2/1
  Add1/1 -> Out_LoR_e/1
  Multiply3/1 -> Add2/1
  Delay5/1 -> Add1/2
  Delay1/1 -> Rate Transition1/1
  Multiply2/1 -> Add1/1
  Delay4/1 -> Add2/2
  Multiply4/1 -> Delay4/1
  Rate Transition2/1 -> Multiply4/2
  In_LoR_e/1 -> Multiply2/2, Delay1/1
  Rate Transition1/1 -> Delay2/1, Multiply3/2
  LoR_4/1 -> Multiply4/1
  LoR_2/1 -> Multiply3/1
  LoR_0/1 -> Multiply2/1

== system coif1_7_Level/3rd_Level_Recon/LoR_Odd1 ==
  In_LoR_o : Inport  OutDataTypeStr=double  SampleTime=1/44100
  Add1 : Sum  AccumDataTypeStr=double  OutDataTypeStr=double  LockScale=on
  Add2 : Sum  AccumDataTypeStr=double  OutDataTypeStr=double  LockScale=on
  Delay{1..2,4..5} (4 alike) : Delay  DelayLength=1  SampleTime=1/44100
  LoR_1 : Constant  Value=0.337897662  OutDataTypeStr=double  SampleTime=1/44100
  LoR_3 : Constant  Value=0.384864847  OutDataTypeStr=double  SampleTime=1/44100
  LoR_5 : Constant  Value=-0.015655728  OutDataTypeStr=double  SampleTime=1/44100
  Multiply2 : Product  OutDataTypeStr=double  LockScale=on
  Multiply3 : Product  OutDataTypeStr=double  LockScale=on
  Multiply4 : Product  OutDataTypeStr=double  LockScale=on
  Rate Transition1 : RateTransition  OutPortSampleTime=1/44100
  Rate Transition2 : RateTransition  OutPortSampleTime=1/44100
  Out_HiR_o : Outport  OutDataTypeStr=double  SampleTime=1/44100  VectorParamsAs1DForOutWhenUnconnected=off
  wires:
  LoR_5/1 -> Multiply4/1
  In_LoR_o/1 -> Multiply2/2, Delay1/1
  LoR_3/1 -> Multiply3/1
  Delay2/1 -> Rate Transition2/1
  Add2/1 -> Delay5/1
  Multiply3/1 -> Add2/1
  Multiply2/1 -> Add1/1
  Delay4/1 -> Add2/2
  Rate Transition1/1 -> Delay2/1, Multiply3/2
  LoR_1/1 -> Multiply2/1
  Delay5/1 -> Add1/2
  Rate Transition2/1 -> Multiply4/2
  Delay1/1 -> Rate Transition1/1
  Multiply4/1 -> Delay4/1
  Add1/1 -> Out_HiR_o/1

== system coif1_7_Level/4th_Level_Decomp/HiD_Even ==
  In_HiD_e : Inport  OutDataTypeStr=double  SampleTime=1/44100
  Add : Sum  AccumDataTypeStr=double  OutDataTypeStr=double  LockScale=on
  Add1 : Sum  AccumDataTypeStr=double  OutDataTypeStr=double  LockScale=on
  Delay{,1..3} (4 alike) : Delay  DelayLength=1  SampleTime=1/44100
  HiD_0 : Constant  Value=0.07273262  OutDataTypeStr=double  SampleTime=1/44100
  HiD_2 : Constant  Value=-0.85257202  OutDataTypeStr=double  SampleTime=1/44100
  HiD_4 : Constant  Value=0.07273262  OutDataTypeStr=double  SampleTime=1/44100
  Multiply : Product  OutDataTypeStr=double  LockScale=on
  Multiply1 : Product  OutDataTypeStr=double  LockScale=on
  Multiply2 : Product  OutDataTypeStr=double  LockScale=on
  Rate Transition : RateTransition  OutPortSampleTime=1/44100
  Rate Transition1 : RateTransition  OutPortSampleTime=1/44100
  Out_HiD_e : Outport  OutDataTypeStr=double  SampleTime=1/44100  VectorParamsAs1DForOutWhenUnconnected=off
  wires:
  In_HiD_e/1 -> Delay/1, Multiply/2
  Delay3/1 -> Add/2
  HiD_2/1 -> Multiply1/1
  Delay/1 -> Rate Transition/1
  Multiply/1 -> Add/1
  Rate Transition/1 -> Delay1/1, Multiply1/2
  HiD_4/1 -> Multiply2/1
  Delay2/1 -> Add1/2
  Multiply1/1 -> Add1/1
  Multiply2/1 -> Delay2/1
  Add1/1 -> Delay3/1
  Rate Transition1/1 -> Multiply2/2
  Add/1 -> Out_HiD_e/1
  Delay1/1 -> Rate Transition1/1
  HiD_0/1 -> Multiply/1

== system coif1_7_Level/4th_Level_Decomp/HiD_Odd ==
  In_HiD_o : Inport  OutDataTypeStr=double  SampleTime=1/44100
  Add : Sum  AccumDataTypeStr=double  OutDataTypeStr=double
  Add1 : Sum  AccumDataTypeStr=double  OutDataTypeStr=double  LockScale=on
  Delay{,1..3} (4 alike) : Delay  DelayLength=1  SampleTime=1/44100
  HiD_1 : Constant  Value=0.337897662  OutDataTypeStr=double  SampleTime=1/44100
  HiD_3 : Constant  Value=0.384864847  OutDataTypeStr=fixdt(1,16,12)  SampleTime=1/44100
  HiD_5 : Constant  Value=-0.015655728  OutDataTypeStr=fixdt(1,16,12)  SampleTime=1/44100
  Multiply : Product  OutDataTypeStr=double  LockScale=on
  Multiply1 : Product  OutDataTypeStr=double  LockScale=on
  Multiply2 : Product  OutDataTypeStr=double  LockScale=on
  Rate Transition : RateTransition  OutPortSampleTime=1/44100
  Rate Transition1 : RateTransition  OutPortSampleTime=1/44100
  Out_HiD_o : Outport  OutDataTypeStr=double  SampleTime=1/44100  VectorParamsAs1DForOutWhenUnconnected=off
  wires:
  In_HiD_o/1 -> Delay/1, Multiply/2
  Delay3/1 -> Add/2
  HiD_3/1 -> Multiply1/1
  Multiply/1 -> Add/1
  Rate Transition/1 -> Delay1/1, Multiply1/2
  Delay2/1 -> Add1/2
  Multiply1/1 -> Add1/1
  Multiply2/1 -> Delay2/1
  Add1/1 -> Delay3/1
  Rate Transition1/1 -> Multiply2/2
  Add/1 -> Out_HiD_o/1
  Delay1/1 -> Rate Transition1/1
  HiD_1/1 -> Multiply/1
  Delay/1 -> Rate Transition/1
  HiD_5/1 -> Multiply2/1

== system coif1_7_Level/4th_Level_Decomp/LoD_Even ==
  In_LoD_e : Inport  OutDataTypeStr=double  SampleTime=1/44100
  Add : Sum  AccumDataTypeStr=double  OutDataTypeStr=double  LockScale=on
  Add1 : Sum  AccumDataTypeStr=double  OutDataTypeStr=double  LockScale=on
  Delay{,1..3} (4 alike) : Delay  DelayLength=1  SampleTime=1/44100
  LoD_0 : Constant  Value=-0.015655728  OutDataTypeStr=double  SampleTime=1/44100
  LoD_2 : Constant  Value=0.384864847  OutDataTypeStr=double  SampleTime=1/44100
  LoD_4 : Constant  Value=0.337897662  OutDataTypeStr=double  SampleTime=1/44100
  Multiply : Product  OutDataTypeStr=double  LockScale=on
  Multiply1 : Product  OutDataTypeStr=double  LockScale=on
  Multiply2 : Product  OutDataTypeStr=double  LockScale=on
  Rate Transition : RateTransition  OutPortSampleTime=1/44100
  Rate Transition1 : RateTransition  OutPortSampleTime=1/44100
  Out_LoD_e : Outport  OutDataTypeStr=double  SampleTime=1/44100  VectorParamsAs1DForOutWhenUnconnected=off
  wires:
  In_LoD_e/1 -> Delay/1, Multiply/2
  Delay3/1 -> Add/2
  LoD_2/1 -> Multiply1/1
  Multiply/1 -> Add/1
  Rate Transition/1 -> Delay1/1, Multiply1/2
  LoD_4/1 -> Multiply2/1
  Delay2/1 -> Add1/2
  Multiply1/1 -> Add1/1
  Multiply2/1 -> Delay2/1
  Add1/1 -> Delay3/1
  Rate Transition1/1 -> Multiply2/2
  Add/1 -> Out_LoD_e/1
  Delay1/1 -> Rate Transition1/1
  LoD_0/1 -> Multiply/1
  Delay/1 -> Rate Transition/1

== system coif1_7_Level/4th_Level_Decomp/LoD_Odd ==
  In_LoD_o : Inport  OutDataTypeStr=double  SampleTime=1/44100
  Add : Sum  AccumDataTypeStr=double  OutDataTypeStr=double  LockScale=on
  Add1 : Sum  AccumDataTypeStr=double  OutDataTypeStr=double  LockScale=on
  Delay{,1..3} (4 alike) : Delay  DelayLength=1  SampleTime=1/44100
  LoD_1 : Constant  Value=-0.07273262  OutDataTypeStr=double  SampleTime=1/44100
  LoD_3 : Constant  Value=0.85257202  OutDataTypeStr=double  SampleTime=1/44100
  LoD_5 : Constant  Value=-0.07273262  OutDataTypeStr=double  SampleTime=1/44100
  Multiply : Product  OutDataTypeStr=double  LockScale=on
  Multiply1 : Product  OutDataTypeStr=double  LockScale=on
  Multiply2 : Product  OutDataTypeStr=double  LockScale=on
  Rate Transition : RateTransition  OutPortSampleTime=1/44100
  Rate Transition1 : RateTransition  OutPortSampleTime=1/44100
  Out_LoD_o : Outport  OutDataTypeStr=double  SampleTime=1/44100  VectorParamsAs1DForOutWhenUnconnected=off
  wires:
  In_LoD_o/1 -> Delay/1, Multiply/2
  Delay3/1 -> Add/2
  LoD_3/1 -> Multiply1/1
  Delay/1 -> Rate Transition/1
  Multiply/1 -> Add/1
  Rate Transition/1 -> Delay1/1, Multiply1/2
  LoD_5/1 -> Multiply2/1
  Delay2/1 -> Add1/2
  Multiply1/1 -> Add1/1
  Multiply2/1 -> Delay2/1
  Add1/1 -> Delay3/1
  Rate Transition1/1 -> Multiply2/2
  Add/1 -> Out_LoD_o/1
  Delay1/1 -> Rate Transition1/1
  LoD_1/1 -> Multiply/1

== system coif1_7_Level/4th_Level_Recon/HiR_Even1 ==
  In_HiR_e : Inport  OutDataTypeStr=double  SampleTime=1/44100
  Add : Sum  AccumDataTypeStr=double  OutDataTypeStr=double  LockScale=on
  Add1 : Sum  AccumDataTypeStr=double  OutDataTypeStr=double  LockScale=on
  Delay{,1..3} (4 alike) : Delay  DelayLength=1  SampleTime=1/44100
  HiR_0 : Constant  Value=-0.015655728  OutDataTypeStr=double  SampleTime=1/44100
  HiR_2 : Constant  Value=0.384864847  OutDataTypeStr=double  SampleTime=1/44100
  HiR_4 : Constant  Value=0.337897662  OutDataTypeStr=double  SampleTime=1/44100
  Multiply : Product  OutDataTypeStr=double  LockScale=on
  Multiply1 : Product  OutDataTypeStr=double  LockScale=on
  Multiply2 : Product  OutDataTypeStr=double  LockScale=on
  Rate Transition : RateTransition  OutPortSampleTime=1/44100
  Rate Transition1 : RateTransition  OutPortSampleTime=1/44100
  Out_HiR_e : Outport  OutDataTypeStr=double  SampleTime=1/44100  VectorParamsAs1DForOutWhenUnconnected=off
  wires:
  In_HiR_e/1 -> Multiply/2, Delay/1
  Delay/1 -> Rate Transition/1
  Delay3/1 -> Add/2
  Multiply/1 -> Add/1
  HiR_0/1 -> Multiply/1
  HiR_2/1 -> Multiply1/1
  Rate Transition/1 -> Delay1/1, Multiply1/2
  Add/1 -> Out_HiR_e/1
  Delay1/1 -> Rate Transition1/1
  Rate Transition1/1 -> Multiply2/2
  Multiply2/1 -> Delay2/1
  Delay2/1 -> Add1/2
  Multiply1/1 -> Add1/1
  Add1/1 -> Delay3/1
  HiR_4/1 -> Multiply2/1

== system coif1_7_Level/4th_Level_Recon/HiR_Odd1 ==
  In_HiR_o : Inport  OutDataTypeStr=double  SampleTime=1/44100
  Add1 : Sum  AccumDataTypeStr=double  OutDataTypeStr=double  LockScale=on
  Add2 : Sum  AccumDataTypeStr=double  OutDataTypeStr=double  LockScale=on
  Delay{1..2,4..5} (4 alike) : Delay  DelayLength=1  SampleTime=1/44100
  HiR_1 : Constant  Value=0.07273262  OutDataTypeStr=double  SampleTime=1/44100
  HiR_3 : Constant  Value=-0.85257202  OutDataTypeStr=double  SampleTime=1/44100
  HiR_5 : Constant  Value=0.07273262  OutDataTypeStr=double  SampleTime=1/44100
  Multiply2 : Product  OutDataTypeStr=double  LockScale=on
  Multiply3 : Product  OutDataTypeStr=double  LockScale=on
  Multiply4 : Product  OutDataTypeStr=double  LockScale=on
  Rate Transition1 : RateTransition  OutPortSampleTime=1/44100
  Rate Transition2 : RateTransition  OutPortSampleTime=1/44100
  Out_HiR_o : Outport  OutDataTypeStr=double  SampleTime=1/44100  VectorParamsAs1DForOutWhenUnconnected=off
  wires:
  HiR_5/1 -> Multiply4/1
  Add1/1 -> Out_HiR_o/1
  Rate Transition2/1 -> Multiply4/2
  Rate Transition1/1 -> Delay2/1, Multiply3/2
  Multiply4/1 -> Delay4/1
  Add2/1 -> Delay5/1
  Multiply3/1 -> Add2/1
  Delay4/1 -> Add2/2
  Multiply2/1 -> Add1/1
  Delay2/1 -> Rate Transition2/1
  In_HiR_o/1 -> Multiply2/2, Delay1/1
  Delay1/1 -> Rate Transition1/1
  Delay5/1 -> Add1/2
  HiR_1/1 -> Multiply2/1
  HiR_3/1 -> Multiply3/1

== system coif1_7_Level/4th_Level_Recon/LoR_Even1 ==
  In_LoR_e : Inport  OutDataTypeStr=double  SampleTime=1/44100
  Add1 : Sum  AccumDataTypeStr=double  OutDataTypeStr=double  LockScale=on
  Add2 : Sum  AccumDataTypeStr=double  OutDataTypeStr=double  LockScale=on
  Delay{1..2,4..5} (4 alike) : Delay  DelayLength=1  SampleTime=1/44100
  LoR_0 : Constant  Value=-0.07273262  OutDataTypeStr=double  SampleTime=1/44100
  LoR_2 : Constant  Value=0.85257202  OutDataTypeStr=double  SampleTime=1/44100
  LoR_4 : Constant  Value=-0.07273262  OutDataTypeStr=double  SampleTime=1/44100
  Multiply2 : Product  OutDataTypeStr=double  LockScale=on
  Multiply3 : Product  OutDataTypeStr=double  LockScale=on
  Multiply4 : Product  OutDataTypeStr=double  LockScale=on
  Rate Transition1 : RateTransition  OutPortSampleTime=1/44100
  Rate Transition2 : RateTransition  OutPortSampleTime=1/44100
  Out_LoR_e : Outport  OutDataTypeStr=double  SampleTime=1/44100  VectorParamsAs1DForOutWhenUnconnected=off
  wires:
  Add2/1 -> Delay5/1
  Delay2/1 -> Rate Transition2/1
  Add1/1 -> Out_LoR_e/1
  Multiply3/1 -> Add2/1
  Delay5/1 -> Add1/2
  Delay1/1 -> Rate Transition1/1
  Multiply2/1 -> Add1/1
  Delay4/1 -> Add2/2
  Multiply4/1 -> Delay4/1
  Rate Transition2/1 -> Multiply4/2
  In_LoR_e/1 -> Multiply2/2, Delay1/1
  Rate Transition1/1 -> Delay2/1, Multiply3/2
  LoR_4/1 -> Multiply4/1
  LoR_2/1 -> Multiply3/1
  LoR_0/1 -> Multiply2/1

== system coif1_7_Level/4th_Level_Recon/LoR_Odd1 ==
  In_LoR_o : Inport  OutDataTypeStr=double  SampleTime=1/44100
  Add1 : Sum  AccumDataTypeStr=double  OutDataTypeStr=double  LockScale=on
  Add2 : Sum  AccumDataTypeStr=double  OutDataTypeStr=double  LockScale=on
  Delay{1..2,4..5} (4 alike) : Delay  DelayLength=1  SampleTime=1/44100
  LoR_1 : Constant  Value=0.337897662  OutDataTypeStr=double  SampleTime=1/44100
  LoR_3 : Constant  Value=0.384864847  OutDataTypeStr=double  SampleTime=1/44100
  LoR_5 : Constant  Value=-0.015655728  OutDataTypeStr=double  SampleTime=1/44100
  Multiply2 : Product  OutDataTypeStr=double  LockScale=on
  Multiply3 : Product  OutDataTypeStr=double  LockScale=on
  Multiply4 : Product  OutDataTypeStr=double  LockScale=on
  Rate Transition1 : RateTransition  OutPortSampleTime=1/44100
  Rate Transition2 : RateTransition  OutPortSampleTime=1/44100
  Out_HiR_o : Outport  OutDataTypeStr=double  SampleTime=1/44100  VectorParamsAs1DForOutWhenUnconnected=off
  wires:
  LoR_5/1 -> Multiply4/1
  In_LoR_o/1 -> Multiply2/2, Delay1/1
  LoR_3/1 -> Multiply3/1
  Delay2/1 -> Rate Transition2/1
  Add2/1 -> Delay5/1
  Multiply3/1 -> Add2/1
  Multiply2/1 -> Add1/1
  Delay4/1 -> Add2/2
  Rate Transition1/1 -> Delay2/1, Multiply3/2
  LoR_1/1 -> Multiply2/1
  Delay5/1 -> Add1/2
  Rate Transition2/1 -> Multiply4/2
  Delay1/1 -> Rate Transition1/1
  Multiply4/1 -> Delay4/1
  Add1/1 -> Out_HiR_o/1

== system coif1_7_Level/5th_Level_Decomp/HiD_Even ==
  In_HiD_e : Inport  OutDataTypeStr=double  SampleTime=1/44100
  Add : Sum  AccumDataTypeStr=double  OutDataTypeStr=double  LockScale=on
  Add1 : Sum  AccumDataTypeStr=double  OutDataTypeStr=double  LockScale=on
  Delay{,1..3} (4 alike) : Delay  DelayLength=1  SampleTime=1/44100
  HiD_0 : Constant  Value=0.07273262  OutDataTypeStr=double  SampleTime=1/44100
  HiD_2 : Constant  Value=-0.85257202  OutDataTypeStr=double  SampleTime=1/44100
  HiD_4 : Constant  Value=0.07273262  OutDataTypeStr=double  SampleTime=1/44100
  Multiply : Product  OutDataTypeStr=double  LockScale=on
  Multiply1 : Product  OutDataTypeStr=double  LockScale=on
  Multiply2 : Product  OutDataTypeStr=double  LockScale=on
  Rate Transition : RateTransition  OutPortSampleTime=1/44100
  Rate Transition1 : RateTransition  OutPortSampleTime=1/44100
  Out_HiD_e : Outport  OutDataTypeStr=double  SampleTime=1/44100  VectorParamsAs1DForOutWhenUnconnected=off
  wires:
  In_HiD_e/1 -> Delay/1, Multiply/2
  Delay3/1 -> Add/2
  HiD_2/1 -> Multiply1/1
  Delay/1 -> Rate Transition/1
  Multiply/1 -> Add/1
  Rate Transition/1 -> Delay1/1, Multiply1/2
  HiD_4/1 -> Multiply2/1
  Delay2/1 -> Add1/2
  Multiply1/1 -> Add1/1
  Multiply2/1 -> Delay2/1
  Add1/1 -> Delay3/1
  Rate Transition1/1 -> Multiply2/2
  Add/1 -> Out_HiD_e/1
  Delay1/1 -> Rate Transition1/1
  HiD_0/1 -> Multiply/1

== system coif1_7_Level/5th_Level_Decomp/HiD_Odd ==
  In_HiD_o : Inport  OutDataTypeStr=double  SampleTime=1/44100
  Add : Sum  AccumDataTypeStr=double  OutDataTypeStr=double
  Add1 : Sum  AccumDataTypeStr=double  OutDataTypeStr=double  LockScale=on
  Delay{,1..3} (4 alike) : Delay  DelayLength=1  SampleTime=1/44100
  HiD_1 : Constant  Value=0.337897662  OutDataTypeStr=double  SampleTime=1/44100
  HiD_3 : Constant  Value=0.384864847  OutDataTypeStr=fixdt(1,16,12)  SampleTime=1/44100
  HiD_5 : Constant  Value=-0.015655728  OutDataTypeStr=fixdt(1,16,12)  SampleTime=1/44100
  Multiply : Product  OutDataTypeStr=double  LockScale=on
  Multiply1 : Product  OutDataTypeStr=double  LockScale=on
  Multiply2 : Product  OutDataTypeStr=double  LockScale=on
  Rate Transition : RateTransition  OutPortSampleTime=1/44100
  Rate Transition1 : RateTransition  OutPortSampleTime=1/44100
  Out_HiD_o : Outport  OutDataTypeStr=double  SampleTime=1/44100  VectorParamsAs1DForOutWhenUnconnected=off
  wires:
  In_HiD_o/1 -> Delay/1, Multiply/2
  Delay3/1 -> Add/2
  HiD_3/1 -> Multiply1/1
  Multiply/1 -> Add/1
  Rate Transition/1 -> Delay1/1, Multiply1/2
  Delay2/1 -> Add1/2
  Multiply1/1 -> Add1/1
  Multiply2/1 -> Delay2/1
  Add1/1 -> Delay3/1
  Rate Transition1/1 -> Multiply2/2
  Add/1 -> Out_HiD_o/1
  Delay1/1 -> Rate Transition1/1
  HiD_1/1 -> Multiply/1
  Delay/1 -> Rate Transition/1
  HiD_5/1 -> Multiply2/1

== system coif1_7_Level/5th_Level_Decomp/LoD_Even ==
  In_LoD_e : Inport  OutDataTypeStr=double  SampleTime=1/44100
  Add : Sum  AccumDataTypeStr=double  OutDataTypeStr=double  LockScale=on
  Add1 : Sum  AccumDataTypeStr=double  OutDataTypeStr=double  LockScale=on
  Delay{,1..3} (4 alike) : Delay  DelayLength=1  SampleTime=1/44100
  LoD_0 : Constant  Value=-0.015655728  OutDataTypeStr=double  SampleTime=1/44100
  LoD_2 : Constant  Value=0.384864847  OutDataTypeStr=double  SampleTime=1/44100
  LoD_4 : Constant  Value=0.337897662  OutDataTypeStr=double  SampleTime=1/44100
  Multiply : Product  OutDataTypeStr=double  LockScale=on
  Multiply1 : Product  OutDataTypeStr=double  LockScale=on
  Multiply2 : Product  OutDataTypeStr=double  LockScale=on
  Rate Transition : RateTransition  OutPortSampleTime=1/44100
  Rate Transition1 : RateTransition  OutPortSampleTime=1/44100
  Out_LoD_e : Outport  OutDataTypeStr=double  SampleTime=1/44100  VectorParamsAs1DForOutWhenUnconnected=off
  wires:
  In_LoD_e/1 -> Delay/1, Multiply/2
  Delay3/1 -> Add/2
  LoD_2/1 -> Multiply1/1
  Multiply/1 -> Add/1
  Rate Transition/1 -> Delay1/1, Multiply1/2
  LoD_4/1 -> Multiply2/1
  Delay2/1 -> Add1/2
  Multiply1/1 -> Add1/1
  Multiply2/1 -> Delay2/1
  Add1/1 -> Delay3/1
  Rate Transition1/1 -> Multiply2/2
  Add/1 -> Out_LoD_e/1
  Delay1/1 -> Rate Transition1/1
  LoD_0/1 -> Multiply/1
  Delay/1 -> Rate Transition/1

== system coif1_7_Level/5th_Level_Decomp/LoD_Odd ==
  In_LoD_o : Inport  OutDataTypeStr=double  SampleTime=1/44100
  Add : Sum  AccumDataTypeStr=double  OutDataTypeStr=double  LockScale=on
  Add1 : Sum  AccumDataTypeStr=double  OutDataTypeStr=double  LockScale=on
  Delay{,1..3} (4 alike) : Delay  DelayLength=1  SampleTime=1/44100
  LoD_1 : Constant  Value=-0.07273262  OutDataTypeStr=double  SampleTime=1/44100
  LoD_3 : Constant  Value=0.85257202  OutDataTypeStr=double  SampleTime=1/44100
  LoD_5 : Constant  Value=-0.07273262  OutDataTypeStr=double  SampleTime=1/44100
  Multiply : Product  OutDataTypeStr=double  LockScale=on
  Multiply1 : Product  OutDataTypeStr=double  LockScale=on
  Multiply2 : Product  OutDataTypeStr=double  LockScale=on
  Rate Transition : RateTransition  OutPortSampleTime=1/44100
  Rate Transition1 : RateTransition  OutPortSampleTime=1/44100
  Out_LoD_o : Outport  OutDataTypeStr=double  SampleTime=1/44100  VectorParamsAs1DForOutWhenUnconnected=off
  wires:
  In_LoD_o/1 -> Delay/1, Multiply/2
  Delay3/1 -> Add/2
  LoD_3/1 -> Multiply1/1
  Delay/1 -> Rate Transition/1
  Multiply/1 -> Add/1
  Rate Transition/1 -> Delay1/1, Multiply1/2
  LoD_5/1 -> Multiply2/1
  Delay2/1 -> Add1/2
  Multiply1/1 -> Add1/1
  Multiply2/1 -> Delay2/1
  Add1/1 -> Delay3/1
  Rate Transition1/1 -> Multiply2/2
  Add/1 -> Out_LoD_o/1
  Delay1/1 -> Rate Transition1/1
  LoD_1/1 -> Multiply/1

== system coif1_7_Level/5th_Level_Recon/HiR_Even1 ==
  In_HiR_e : Inport  OutDataTypeStr=double  SampleTime=1/44100
  Add : Sum  AccumDataTypeStr=double  OutDataTypeStr=double  LockScale=on
  Add1 : Sum  AccumDataTypeStr=double  OutDataTypeStr=double  LockScale=on
  Delay{,1..3} (4 alike) : Delay  DelayLength=1  SampleTime=1/44100
  HiR_0 : Constant  Value=-0.015655728  OutDataTypeStr=double  SampleTime=1/44100
  HiR_2 : Constant  Value=0.384864847  OutDataTypeStr=double  SampleTime=1/44100
  HiR_4 : Constant  Value=0.337897662  OutDataTypeStr=double  SampleTime=1/44100
  Multiply : Product  OutDataTypeStr=double  LockScale=on
  Multiply1 : Product  OutDataTypeStr=double  LockScale=on
  Multiply2 : Product  OutDataTypeStr=double  LockScale=on
  Rate Transition : RateTransition  OutPortSampleTime=1/44100
  Rate Transition1 : RateTransition  OutPortSampleTime=1/44100
  Out_HiR_e : Outport  OutDataTypeStr=double  SampleTime=1/44100  VectorParamsAs1DForOutWhenUnconnected=off
  wires:
  In_HiR_e/1 -> Multiply/2, Delay/1
  Delay/1 -> Rate Transition/1
  Delay3/1 -> Add/2
  Multiply/1 -> Add/1
  HiR_0/1 -> Multiply/1
  HiR_2/1 -> Multiply1/1
  Rate Transition/1 -> Delay1/1, Multiply1/2
  Add/1 -> Out_HiR_e/1
  Delay1/1 -> Rate Transition1/1
  Rate Transition1/1 -> Multiply2/2
  Multiply2/1 -> Delay2/1
  Delay2/1 -> Add1/2
  Multiply1/1 -> Add1/1
  Add1/1 -> Delay3/1
  HiR_4/1 -> Multiply2/1
